simulink model "SWC_VES_type"  (R2021b)
settings: Solver=FixedStepDiscrete  StartTime=0.0  StopTime=10.0  FixedStep=0.001  RelTol=1e-3
undefined symbols (not defined in the file or in its folder): R_HALINCDD_CSOP_IPCF_Handler
libraries: simulink x32
settings Model: DataDictionary=APPTypes.sldd  Creator=FVT23010  LastModifiedBy=FVT23010
settings DataIOCC: SaveFormat=StructureWithTime
settings OptimizationCC: DefaultParameterBehavior=Inlined  EnhancedBackFolding=on  PassReuseOutputArgsAs=Individual arguments  ZeroExternalMemoryAtStartup=off  ZeroInternalMemoryAtStartup=off  OptimizeBlockOrder=speed  DifferentSizesBufferReuse=on  OptimizationCustomize=off  EfficientTunableParamExpr=on
settings DebuggingCC: ParameterTunabilityLossMsg=error
settings HardwareCC: ProdBitPerPointer=32  ProdBitPerSizeT=32  ProdBitPerPtrDiffT=32  ProdLargestAtomicInteger=Long  ProdLargestAtomicFloat=Double  ProdWordSize=32  ProdLongLongMode=on  ProdHWDeviceType=ARM Compatible->ARM Cortex-M
settings ModelReferenceCC: ModelReferenceNumInstancesAllowed=Single
settings SFSimCC: MATLABDynamicMemAlloc=off
settings RTWCC: Description=AUTOSAR  SystemTargetFile=autosar.tlc  GenCodeOnly=on  TemplateMakefile=ert_default_tmf  PortableWordSizes=on
settings CodeAppCC: ForceParamTrailComments=on  IgnoreCustomStorageClasses=off  OperatorAnnotations=on  SimulinkDataObjDesc=on  SFDataObjDesc=on  InsertBlockDesc=on
settings STFCustomTargetCC: TargetLangStandard=C99 (ISO)  MultiwordLength=256  ParMdlRefBuildCompliant=on  CompOptLevelCompliant=on  IncludeMdlTerminateFcn=off  CombineOutputUpdateFcns=on  SuppressErrorStatus=on  ERTCustomFileBanners=on  SupportNonFinite=off  SupportComplex=off  SupportContinuousTime=off  SupportNonInlinedSFcns=off  RemoveResetFunc=on  MATLABClassNameForMDSCustomization=Simulink.SoftwareTarget.ERTCustomization  AutosarCompliant=on  GRTInterface=off  UseToolchainInfoCompliant=on  LookupTableObjectStructAxisOrder=2,1,3,4,...  LUTObjectStructOrderEvenSpacing=Size,Table,Breakpoints  SystemTargetFile=autosar.tlc
settings ERTTargetCC: TargetLangStandard=C99 (ISO)  ConcurrentExecutionCompliant=off  IncludeMdlTerminateFcn=off  SuppressErrorStatus=on  SupportNonFinite=off  SupportComplex=off  ModelStepFunctionPrototypeControlCompliant=off  CPPClassGenCompliant=off  AutosarCompliant=on  LookupTableObjectStructAxisOrder=2,1,3,4,...  LUTObjectStructOrderEvenSpacing=Size,Table,Breakpoints  GenerateASAP2=on  InlinedParameterPlacement=NonHierarchical  ERTCustomFileTemplate=example_file_process.tlc  ConvertIfToSwitch=off  SuppressUnreachableDefaultCases=off  BooleanTrueId=true_MatlabRTW  BooleanFalseId=false_MatlabRTW

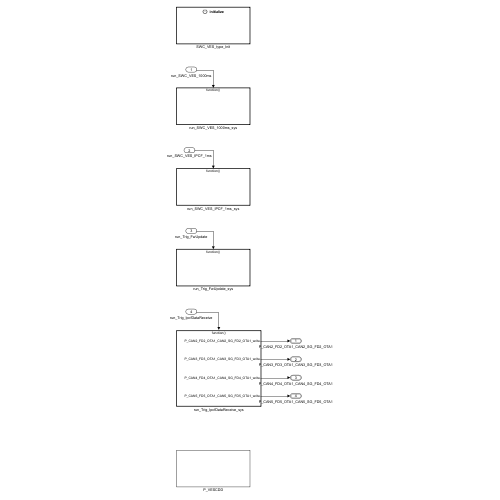
[thumbnail: Simulink's stored preview of the top-level diagram]
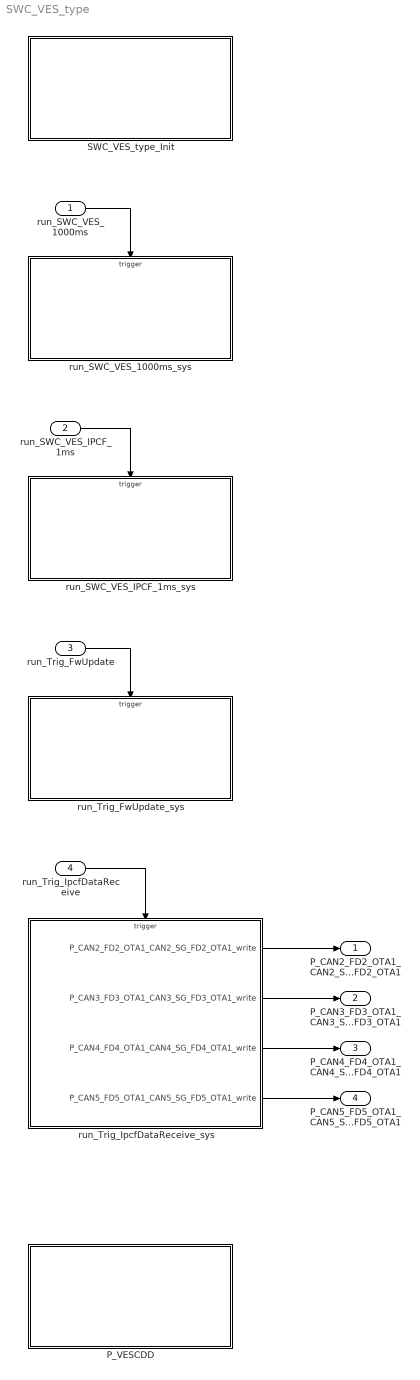
== system SWC_VES_type ==
  run_SWC_VES_1000ms : Inport  SampleTime=1  OutputFunctionCall=on
  run_SWC_VES_IPCF_1ms : Inport  Port=2  SampleTime=0.001  OutputFunctionCall=on
  run_Trig_FwUpdate : Inport  Port=3  OutputFunctionCall=on
  run_Trig_IpcfDataReceive : Inport  Port=4  OutputFunctionCall=on
  P_VESCDD : Subsystem
  SWC_VES_type_Init : Subsystem
  run_SWC_VES_1000ms_sys : Subsystem
  run_SWC_VES_IPCF_1ms_sys : Subsystem
  run_Trig_FwUpdate_sys : Subsystem
  run_Trig_IpcfDataReceive_sys : Subsystem
  P_CAN2_FD2_OTA1_CAN2_SG_FD2_OTA1 : Outport  OutDataTypeStr=Bus: DT_CAN2_SG_FD2_OTA1  PortDimensions=1  BusOutputAsStruct=on
  P_CAN3_FD3_OTA1_CAN3_SG_FD3_OTA1 : Outport  Port=2  OutDataTypeStr=Bus: DT_CAN3_SG_FD3_OTA1  PortDimensions=1  BusOutputAsStruct=on
  P_CAN4_FD4_OTA1_CAN4_SG_FD4_OTA1 : Outport  Port=3  OutDataTypeStr=Bus: DT_CAN4_SG_FD4_OTA1  PortDimensions=1  BusOutputAsStruct=on
  P_CAN5_FD5_OTA1_CAN5_SG_FD5_OTA1 : Outport  Port=4  OutDataTypeStr=Bus: DT_CAN5_SG_FD5_OTA1  PortDimensions=1  BusOutputAsStruct=on
  wires:
  run_Trig_IpcfDataReceive_sys/1(P_CAN2_FD2_OTA1_CAN2_SG_FD2_OTA1_write) -> P_CAN2_FD2_OTA1_CAN2_SG_FD2_OTA1/1
  run_Trig_IpcfDataReceive_sys/2(P_CAN3_FD3_OTA1_CAN3_SG_FD3_OTA1_write) -> P_CAN3_FD3_OTA1_CAN3_SG_FD3_OTA1/1
  run_Trig_IpcfDataReceive_sys/3(P_CAN4_FD4_OTA1_CAN4_SG_FD4_OTA1_write) -> P_CAN4_FD4_OTA1_CAN4_SG_FD4_OTA1/1
  run_Trig_IpcfDataReceive_sys/4(P_CAN5_FD5_OTA1_CAN5_SG_FD5_OTA1_write) -> P_CAN5_FD5_OTA1_CAN5_SG_FD5_OTA1/1
  run_SWC_VES_1000ms/1 -> run_SWC_VES_1000ms_sys/Trigger
  run_SWC_VES_IPCF_1ms/1 -> run_SWC_VES_IPCF_1ms_sys/Trigger
  run_Trig_FwUpdate/1 -> run_Trig_FwUpdate_sys/Trigger
  run_Trig_IpcfDataReceive/1 -> run_Trig_IpcfDataReceive_sys/Trigger

== system SWC_VES_type/P_VESCDD ==
  run_VESCDD_sys : Subsystem

== system SWC_VES_type/SWC_VES_type_Init ==
  Event Listener : EventListener  EventName=reset

== system SWC_VES_type/run_SWC_VES_1000ms_sys ==
  function : TriggerPort  TriggerType=function-call  VariantControl=(inherit)  SampleTimeType=periodic  SampleTime=-1

== system SWC_VES_type/run_SWC_VES_IPCF_1ms_sys ==
  function : TriggerPort  TriggerType=function-call  VariantControl=(inherit)  SampleTimeType=periodic  SampleTime=-1
  R_HALINCDD_CSOP_IPCF_Handler : FunctionCaller  FunctionPrototype=R_HALINCDD_CSOP_IPCF_Handler()

== system SWC_VES_type/run_Trig_FwUpdate_sys ==
  function : TriggerPort  TriggerType=function-call  VariantControl=(inherit)

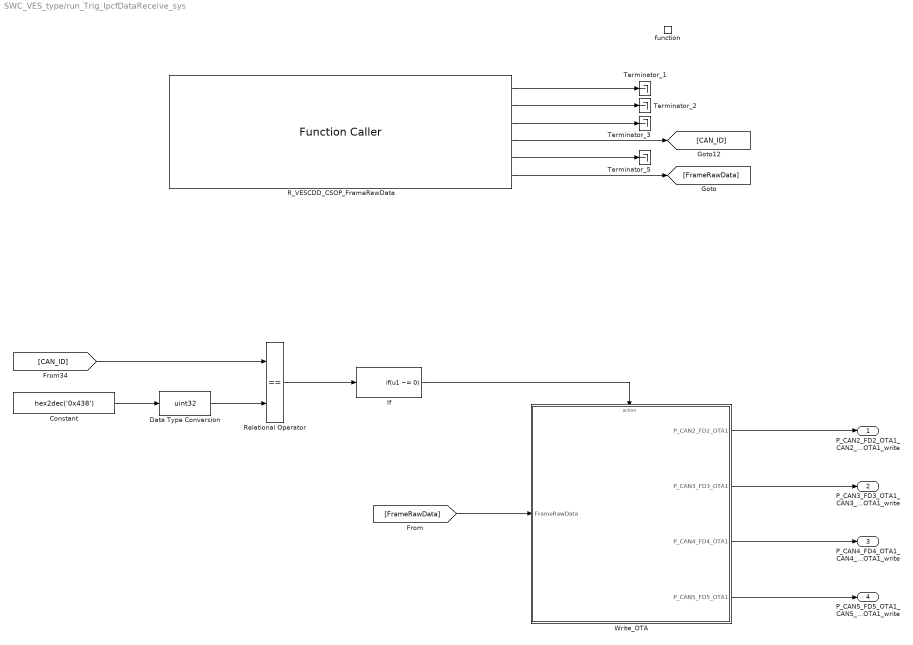
== system SWC_VES_type/run_Trig_IpcfDataReceive_sys ==
  function : TriggerPort  TriggerType=function-call  VariantControl=(inherit)
  Constant : Constant  Value=hex2dec('0x438')
  Data Type Conversion : DataTypeConversion  OutDataTypeStr=uint32
  If : If  IfExpression=u1 ~= 0  ShowElse=off
  R_VESCDD_CSOP_FrameRawData : FunctionCaller  FunctionPrototype=[channel,fd,ext,id,dlc,FrameRawData] = R_VESCDD_CSOP_FrameRawData()  OutputArgumentSpecifications=uint8(1), uint8(1), uint8(1), uint32(1), uint8(1), uint8([1;1;1;1;1;1;1;1;1;1;1;1;1;1;1;1;1;1;1;1;1;1;1;1;1;1;1;1;1;1;1;1;1;1;1;1;1;1;1;1;1;1;1;1;1;1;1;1;1;1;1;1;1;1;1;1;1;1;1;1;1;1;1;1])
  Relational Operator : RelationalOperator  Operator===  OutDataTypeStr=boolean  RndMeth=Simplest
  Terminator_{1..3,5} (4 alike) : Terminator
  Write_OTA : Subsystem  TreatAsAtomicUnit=on
  P_CAN2_FD2_OTA1_CAN2_SG_FD2_OTA1_write : Outport
  P_CAN3_FD3_OTA1_CAN3_SG_FD3_OTA1_write : Outport  Port=2
  P_CAN4_FD4_OTA1_CAN4_SG_FD4_OTA1_write : Outport  Port=3
  P_CAN5_FD5_OTA1_CAN5_SG_FD5_OTA1_write : Outport  Port=4
  wires:
  R_VESCDD_CSOP_FrameRawData/6 -> [FrameRawData]
  R_VESCDD_CSOP_FrameRawData/3 -> Terminator_3/1
  R_VESCDD_CSOP_FrameRawData/5 -> Terminator_5/1
  R_VESCDD_CSOP_FrameRawData/4 -> [CAN_ID]
  R_VESCDD_CSOP_FrameRawData/1 -> Terminator_1/1
  R_VESCDD_CSOP_FrameRawData/2 -> Terminator_2/1
  [FrameRawData] -> Write_OTA/1(FrameRawData)
  Relational Operator/1 -> If/1
  [CAN_ID] -> Relational Operator/1
  Constant/1 -> Data Type Conversion/1
  If/1 -> Write_OTA/Action
  Data Type Conversion/1 -> Relational Operator/2
  Write_OTA/1(P_CAN2_FD2_OTA1) -> P_CAN2_FD2_OTA1_CAN2_SG_FD2_OTA1_write/1
  Write_OTA/2(P_CAN3_FD3_OTA1) -> P_CAN3_FD3_OTA1_CAN3_SG_FD3_OTA1_write/1
  Write_OTA/3(P_CAN4_FD4_OTA1) -> P_CAN4_FD4_OTA1_CAN4_SG_FD4_OTA1_write/1
  Write_OTA/4(P_CAN5_FD5_OTA1) -> P_CAN5_FD5_OTA1_CAN5_SG_FD5_OTA1_write/1

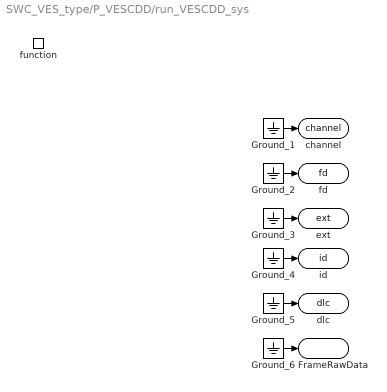
== system SWC_VES_type/P_VESCDD/run_VESCDD_sys ==
  function : TriggerPort  TriggerType=function-call  IsSimulinkFunction=on  FunctionName=run_VESCDD  VariantControl=(inherit)
  Ground_{1..6} (6 alike) : Ground
  channel : ArgOut  OutDataTypeStr=uint8  ArgumentName=channel
  fd : ArgOut  Port=2  OutDataTypeStr=uint8  ArgumentName=fd
  ext : ArgOut  Port=3  OutDataTypeStr=uint8  ArgumentName=ext
  id : ArgOut  Port=4  OutDataTypeStr=uint32  ArgumentName=id
  dlc : ArgOut  Port=5  OutDataTypeStr=uint8  ArgumentName=dlc
  FrameRawData : ArgOut  Port=6  OutDataTypeStr=uint8  PortDimensions=64  ArgumentName=FrameRawData
  wires:
  Ground_1/1 -> channel/1
  Ground_2/1 -> fd/1
  Ground_3/1 -> ext/1
  Ground_4/1 -> id/1
  Ground_5/1 -> dlc/1
  Ground_6/1 -> FrameRawData/1

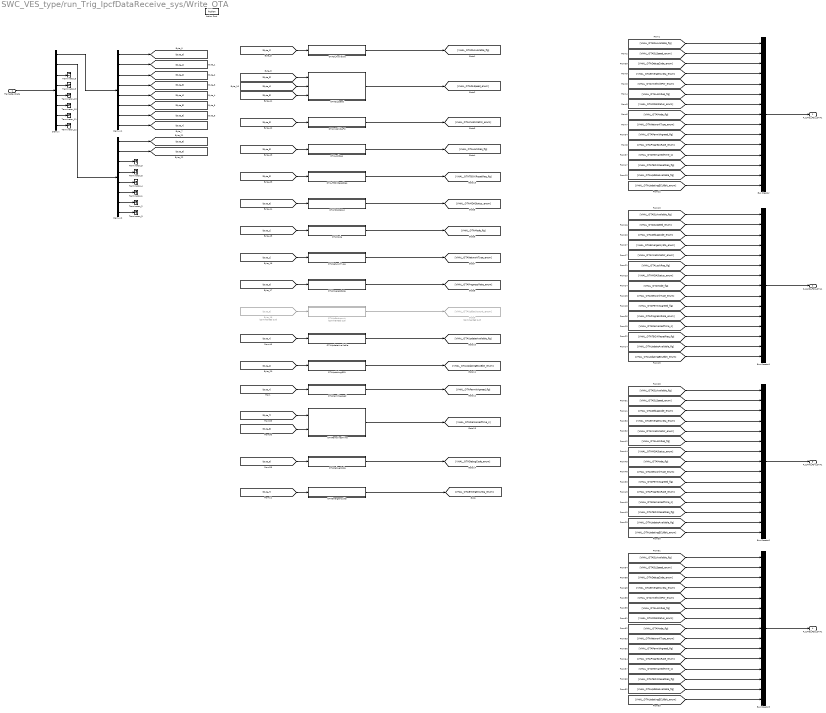
== system SWC_VES_type/run_Trig_IpcfDataReceive_sys/Write_OTA ==
  FrameRawData : Inport
  Action Port : ActionPort  ActionPortLabel=if(u1 ~= 0)
  Bus Creator : BusCreator  Inputs=15  OutDataTypeStr=Bus: DT_CAN2_SG_FD2_OTA1  NonVirtualBus=on
      settings: InheritFromInputs=off
  Bus Creator1 : BusCreator  Inputs=15  OutDataTypeStr=Bus: DT_CAN3_SG_FD3_OTA1  NonVirtualBus=on
      settings: InheritFromInputs=off
  Bus Creator2 : BusCreator  Inputs=15  OutDataTypeStr=Bus: DT_CAN4_SG_FD4_OTA1  NonVirtualBus=on
      settings: InheritFromInputs=off
  Bus Creator3 : BusCreator  Inputs=15  OutDataTypeStr=Bus: DT_CAN5_SG_FD5_OTA1  NonVirtualBus=on
      settings: InheritFromInputs=off
  Byte_18 : From  Commented=on  GotoTag=Byte_6
  Demux : Demux  Outputs=8
  Demux1 : Demux  Outputs=8
  Demux2 : Demux  Outputs=8
  Goto9 : Goto  Commented=on  GotoTag=VHAL_OTAUpBackcount_enum
  OTADLAvailable : Subsystem
  OTADLSpeed : Subsystem
  OTADebugCode : Subsystem
  OTAEmergencySta : Subsystem
  OTAInVehicleFW : Subsystem
  OTALockReq : Subsystem
  OTAMDAStatus : Subsystem
  OTAMode : Subsystem
  OTANetworkType : Subsystem
  OTAPermitAgreed : Subsystem
  OTAProgressRate : Subsystem
  OTARemainedTime : Subsystem
  OTAUpBackcount : Subsystem  Commented=on
  OTAUpdateAvailable : Subsystem
  OTAUpdatingECU : Subsystem
  OTA_TBOXResetReq : Subsystem
  Terminator_{1..6,8..13} (12 alike) : Terminator
  P_CAN2_FD2_OTA1 : Outport
  P_CAN3_FD3_OTA1 : Outport  Port=2
  P_CAN4_FD4_OTA1 : Outport  Port=3
  P_CAN5_FD5_OTA1 : Outport  Port=4
  wires:
  [Byte_2] -> OTAUpdatingECU/1(Byte_2)
  Demux1/7 -> [Byte_6]  "Raw_Byte6"
  Demux1/4 -> [Byte_3]  "Raw_Byte3"
  Demux1/6 -> [Byte_5]  "Raw_Byte5"
  [Byte_5] -> OTADLSpeed/3(Byte_5)
  Demux/1 -> Demux1/1
  [Byte_7] -> OTAUpdateAvailable/1(Byte_7)
  Demux/4 -> Terminator_9/1
  [Byte_3] -> OTALockReq/1(Byte_3)
  [Byte_3] -> OTADLSpeed/1(Byte_3)
  Demux/5 -> Terminator_13/1
  [Byte_4] -> OTADLSpeed/2(Byte_4)
  Byte_18/1 -> OTAUpBackcount/1(Byte_6)
  Demux1/8 -> [Byte_7]  "Raw_Byte7"
  Demux1/3 -> [Byte_2]  "Raw_Byte2"
  Demux1/2 -> [Byte_1]  "Raw_Byte1"
  Demux1/5 -> [Byte_4]  "Raw_Byte4"
  Demux1/1 -> [Byte_0]  "Raw_Byte0"
  [Byte_1] -> OTANetworkType/1(Byte_1)
  Demux/7 -> Terminator_11/1
  FrameRawData/1 -> Demux/1
  [Byte_6] -> OTAMDAStatus/1(Byte_1)
  Demux/3 -> Terminator_8/1
  [Byte_1] -> OTAMode/1(Byte_1)
  [Byte_0] -> OTAProgressRate/1(Byte_0)
  [Byte_3] -> OTAInVehicleFW/1(Byte_3)
  [Byte_1] -> OTADLAvailable/1(Byte_1)
  Demux/8 -> Terminator_12/1
  Demux/6 -> Terminator_10/1
  OTAUpdateAvailable/1(VHAL_OTAUpdateAvailable_flg) -> [VHAL_OTAUpdateAvailable_flg]
  OTAMode/1(VHAL_OTAMode_flg) -> [VHAL_OTAMode_flg]
  OTAInVehicleFW/1(VHAL_OTAInVehicleFW_enum) -> [VHAL_OTAInVehicleFW_enum]
  OTADLAvailable/1(VHAL_OTADLAvailable_flg) -> [VHAL_OTADLAvailable_flg]
  OTANetworkType/1(VHAL_OTANetworkType_enum) -> [VHAL_OTANetworkType_enum]
  OTADLSpeed/1(VHAL_OTADLSpeed_enum) -> [VHAL_OTADLSpeed_enum]
  OTAMDAStatus/1(VHAL_OTAMDAStatus_enum) -> [VHAL_OTAMDAStatus_enum]
  OTAUpdatingECU/1(VHAL_OTAUpdatingECU_enum) -> [VHAL_OTAUpdatingECU8bit_enum]
  OTALockReq/1(VHAL_OTALockReq_flg) -> [VHAL_OTALockReq_flg]
  OTAUpBackcount/1(VHAL_OTAUpBackcount_enum) -> Goto9/1
  OTAProgressRate/1(VHAL_OTAProgressRate_enum) -> [VHAL_OTAProgressRate_enum]
  Demux/2 -> Demux2/1
  Demux2/1 -> [Byte_8]  "Raw_Byte8"
  Demux2/2 -> [Byte_9]  "Raw_Byte9"
  Demux2/3 -> Terminator_5/1
  Demux2/5 -> Terminator_4/1
  Demux2/6 -> Terminator_1/1
  Demux2/7 -> Terminator_2/1
  Demux2/8 -> Terminator_3/1
  [Byte_7] -> OTAPermitAgreed/1(Byte_7)
  OTAPermitAgreed/1(VHAL_OTAPermitAgreed_flg) -> [VHAL_OTAPermitAgreed_flg]
  [Byte_8] -> OTARemainedTime/2(Byte_8)
  [Byte_7] -> OTARemainedTime/1(Byte_7)
  OTARemainedTime/1(VHAL_OTARemainedTime_s) -> [VHAL_OTARemainedTime_s]
  [Byte_9] -> OTADebugCode/1(Byte_9)
  OTADebugCode/1(VHAL_OTADebugCode_enum) -> [VHAL_OTADebugCode_enum]
  [VHAL_OTADLAvailable_flg] -> Bus Creator/1
  [VHAL_OTADebugCode_enum] -> Bus Creator/3
  Bus Creator/1 -> P_CAN2_FD2_OTA1/1
  [VHAL_OTADLSpeed_enum] -> Bus Creator/2
  Demux2/4 -> Terminator_6/1  "Raw_Byte11"
  OTA_TBOXResetReq/1(VHAL_OTALockReq_flg) -> [VHAL_OTATBOXResetReq_flg]
  [Byte_3] -> OTA_TBOXResetReq/1(Byte_3)
  [VHAL_OTAEmergencySta_enum] -> Bus Creator/4
  [VHAL_OTAInVehicleFW_enum] -> Bus Creator/5
  [VHAL_OTALockReq_flg] -> Bus Creator/6
  [VHAL_OTAMDAStatus_enum] -> Bus Creator/7
  [VHAL_OTAMode_flg] -> Bus Creator/8
  [VHAL_OTANetworkType_enum] -> Bus Creator/9
  [VHAL_OTAPermitAgreed_flg] -> Bus Creator/10
  [VHAL_OTAProgressRate_enum] -> Bus Creator/11
  [VHAL_OTARemainedTime_s] -> Bus Creator/12
  [VHAL_OTATBOXResetReq_flg] -> Bus Creator/13
  [VHAL_OTAUpdateAvailable_flg] -> Bus Creator/14
  [VHAL_OTAUpdatingECU8bit_enum] -> Bus Creator/15
  OTAEmergencySta/1(VHAL_OTAEmergencySta_enum) -> [VHAL_OTAEmergencySta_enum]
  [Byte_7] -> OTAEmergencySta/1(Byte_7)
  [VHAL_OTAUpdatingECU8bit_enum] -> Bus Creator1/15
  [VHAL_OTAUpdateAvailable_flg] -> Bus Creator1/14
  [VHAL_OTATBOXResetReq_flg] -> Bus Creator1/13
  [VHAL_OTARemainedTime_s] -> Bus Creator1/12
  [VHAL_OTAProgressRate_enum] -> Bus Creator1/11
  [VHAL_OTAPermitAgreed_flg] -> Bus Creator1/10
  [VHAL_OTANetworkType_enum] -> Bus Creator1/9
  [VHAL_OTAMode_flg] -> Bus Creator1/8
  [VHAL_OTAMDAStatus_enum] -> Bus Creator1/7
  [VHAL_OTALockReq_flg] -> Bus Creator1/6
  [VHAL_OTAInVehicleFW_enum] -> Bus Creator1/5
  [VHAL_OTAEmergencySta_enum] -> Bus Creator1/4
  [VHAL_OTADLSpeed_enum] -> Bus Creator1/2
  Bus Creator1/1 -> P_CAN3_FD3_OTA1/1
  [VHAL_OTADebugCode_enum] -> Bus Creator1/3
  [VHAL_OTADLAvailable_flg] -> Bus Creator1/1
  [VHAL_OTADLAvailable_flg] -> Bus Creator2/1
  [VHAL_OTADebugCode_enum] -> Bus Creator2/3
  Bus Creator2/1 -> P_CAN4_FD4_OTA1/1
  [VHAL_OTADLSpeed_enum] -> Bus Creator2/2
  [VHAL_OTAEmergencySta_enum] -> Bus Creator2/4
  [VHAL_OTAInVehicleFW_enum] -> Bus Creator2/5
  [VHAL_OTALockReq_flg] -> Bus Creator2/6
  [VHAL_OTAMDAStatus_enum] -> Bus Creator2/7
  [VHAL_OTAMode_flg] -> Bus Creator2/8
  [VHAL_OTANetworkType_enum] -> Bus Creator2/9
  [VHAL_OTAPermitAgreed_flg] -> Bus Creator2/10
  [VHAL_OTAProgressRate_enum] -> Bus Creator2/11
  [VHAL_OTARemainedTime_s] -> Bus Creator2/12
  [VHAL_OTATBOXResetReq_flg] -> Bus Creator2/13
  [VHAL_OTAUpdateAvailable_flg] -> Bus Creator2/14
  [VHAL_OTAUpdatingECU8bit_enum] -> Bus Creator2/15
  [VHAL_OTAUpdatingECU8bit_enum] -> Bus Creator3/15
  [VHAL_OTAUpdateAvailable_flg] -> Bus Creator3/14
  [VHAL_OTATBOXResetReq_flg] -> Bus Creator3/13
  [VHAL_OTARemainedTime_s] -> Bus Creator3/12
  [VHAL_OTAProgressRate_enum] -> Bus Creator3/11
  [VHAL_OTAPermitAgreed_flg] -> Bus Creator3/10
  [VHAL_OTANetworkType_enum] -> Bus Creator3/9
  [VHAL_OTAMode_flg] -> Bus Creator3/8
  [VHAL_OTAMDAStatus_enum] -> Bus Creator3/7
  [VHAL_OTALockReq_flg] -> Bus Creator3/6
  [VHAL_OTAInVehicleFW_enum] -> Bus Creator3/5
  [VHAL_OTAEmergencySta_enum] -> Bus Creator3/4
  [VHAL_OTADLSpeed_enum] -> Bus Creator3/2
  Bus Creator3/1 -> P_CAN5_FD5_OTA1/1
  [VHAL_OTADebugCode_enum] -> Bus Creator3/3
  [VHAL_OTADLAvailable_flg] -> Bus Creator3/1

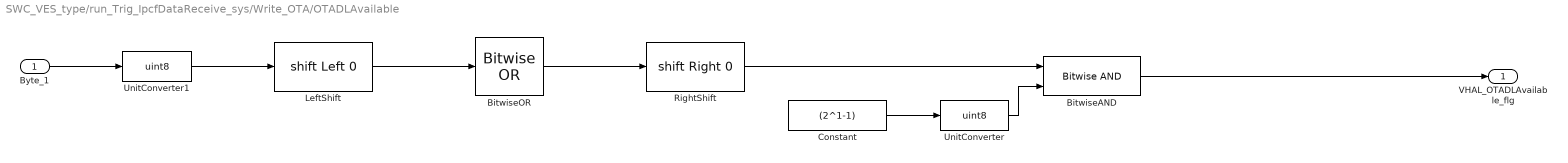
== system SWC_VES_type/run_Trig_IpcfDataReceive_sys/Write_OTA/OTADLAvailable ==
  Byte_1 : Inport
  BitwiseAND : simulink/Logic and Bit Operations/Bitwise Operator  logicop=AND  UseBitMask=off  NumInputPorts=2  BitMask=bin2dec('11011001')  BitMaskRealWorld=Stored Integer
  BitwiseOR : simulink/Logic and Bit Operations/Bitwise Operator  logicop=OR  UseBitMask=off  BitMask=bin2dec('11011001')  BitMaskRealWorld=Stored Integer
  Constant : Constant  Value=(2^1-1)
  LeftShift : ArithShift  BitShiftDirection=Left
  RightShift : ArithShift  BitShiftDirection=Right
  UnitConverter : DataTypeConversion  OutDataTypeStr=uint8
  UnitConverter1 : DataTypeConversion  OutDataTypeStr=uint8
  VHAL_OTADLAvailable_flg : Outport
  wires:
  BitwiseOR/1 -> RightShift/1
  RightShift/1 -> BitwiseAND/1
  UnitConverter/1 -> BitwiseAND/2
  Constant/1 -> UnitConverter/1
  BitwiseAND/1 -> VHAL_OTADLAvailable_flg/1
  LeftShift/1 -> BitwiseOR/1
  UnitConverter1/1 -> LeftShift/1
  Byte_1/1 -> UnitConverter1/1

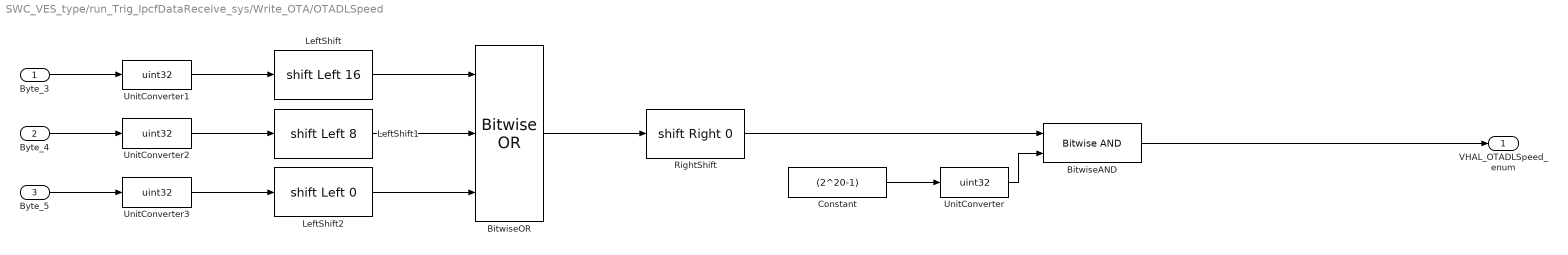
== system SWC_VES_type/run_Trig_IpcfDataReceive_sys/Write_OTA/OTADLSpeed ==
  Byte_3 : Inport
  Byte_4 : Inport  Port=2
  Byte_5 : Inport  Port=3
  BitwiseAND : simulink/Logic and Bit Operations/Bitwise Operator  logicop=AND  UseBitMask=off  NumInputPorts=2  BitMask=bin2dec('11011001')  BitMaskRealWorld=Stored Integer
  BitwiseOR : simulink/Logic and Bit Operations/Bitwise Operator  logicop=OR  UseBitMask=off  NumInputPorts=3  BitMask=bin2dec('11011001')  BitMaskRealWorld=Stored Integer
  Constant : Constant  Value=(2^20-1)
  LeftShift : ArithShift  BitShiftNumber=16  BitShiftDirection=Left
  LeftShift1 : ArithShift  BitShiftNumber=8  BitShiftDirection=Left
  LeftShift2 : ArithShift  BitShiftDirection=Left
  RightShift : ArithShift  BitShiftDirection=Right
  UnitConverter{,1..3} (4 alike) : DataTypeConversion  OutDataTypeStr=uint32
  VHAL_OTADLSpeed_enum : Outport
  wires:
  BitwiseOR/1 -> RightShift/1
  RightShift/1 -> BitwiseAND/1
  UnitConverter/1 -> BitwiseAND/2
  Constant/1 -> UnitConverter/1
  BitwiseAND/1 -> VHAL_OTADLSpeed_enum/1
  LeftShift/1 -> BitwiseOR/1
  UnitConverter1/1 -> LeftShift/1
  Byte_3/1 -> UnitConverter1/1
  LeftShift1/1 -> BitwiseOR/2
  UnitConverter2/1 -> LeftShift1/1
  Byte_4/1 -> UnitConverter2/1
  LeftShift2/1 -> BitwiseOR/3
  UnitConverter3/1 -> LeftShift2/1
  Byte_5/1 -> UnitConverter3/1

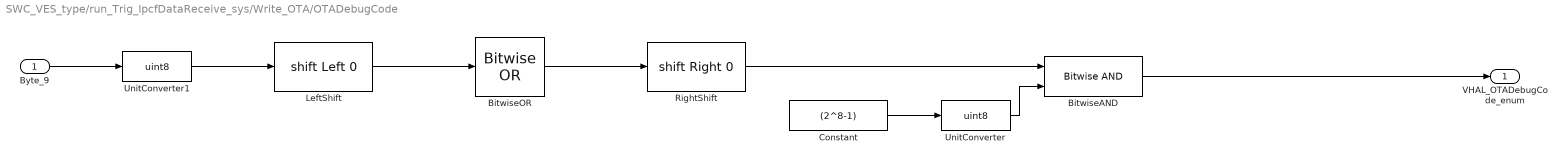
== system SWC_VES_type/run_Trig_IpcfDataReceive_sys/Write_OTA/OTADebugCode ==
  Byte_9 : Inport
  BitwiseAND : simulink/Logic and Bit Operations/Bitwise Operator  logicop=AND  UseBitMask=off  NumInputPorts=2  BitMask=bin2dec('11011001')  BitMaskRealWorld=Stored Integer
  BitwiseOR : simulink/Logic and Bit Operations/Bitwise Operator  logicop=OR  UseBitMask=off  BitMask=bin2dec('11011001')  BitMaskRealWorld=Stored Integer
  Constant : Constant  Value=(2^8-1)
  LeftShift : ArithShift  BitShiftDirection=Left
  RightShift : ArithShift  BitShiftDirection=Right
  UnitConverter : DataTypeConversion  OutDataTypeStr=uint8
  UnitConverter1 : DataTypeConversion  OutDataTypeStr=uint8
  VHAL_OTADebugCode_enum : Outport
  wires:
  BitwiseOR/1 -> RightShift/1
  RightShift/1 -> BitwiseAND/1
  UnitConverter/1 -> BitwiseAND/2
  Constant/1 -> UnitConverter/1
  BitwiseAND/1 -> VHAL_OTADebugCode_enum/1
  LeftShift/1 -> BitwiseOR/1
  UnitConverter1/1 -> LeftShift/1
  Byte_9/1 -> UnitConverter1/1

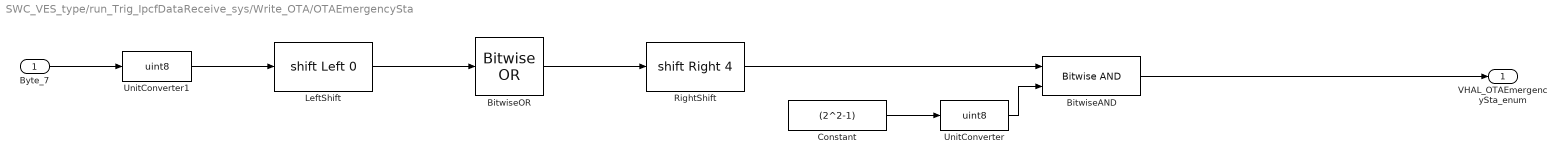
== system SWC_VES_type/run_Trig_IpcfDataReceive_sys/Write_OTA/OTAEmergencySta ==
  Byte_7 : Inport
  BitwiseAND : simulink/Logic and Bit Operations/Bitwise Operator  logicop=AND  UseBitMask=off  NumInputPorts=2  BitMask=bin2dec('11011001')  BitMaskRealWorld=Stored Integer
  BitwiseOR : simulink/Logic and Bit Operations/Bitwise Operator  logicop=OR  UseBitMask=off  BitMask=bin2dec('11011001')  BitMaskRealWorld=Stored Integer
  Constant : Constant  Value=(2^2-1)
  LeftShift : ArithShift  BitShiftDirection=Left
  RightShift : ArithShift  BitShiftNumber=4  BitShiftDirection=Right
  UnitConverter : DataTypeConversion  OutDataTypeStr=uint8
  UnitConverter1 : DataTypeConversion  OutDataTypeStr=uint8
  VHAL_OTAEmergencySta_enum : Outport
  wires:
  Byte_7/1 -> UnitConverter1/1
  UnitConverter1/1 -> LeftShift/1
  LeftShift/1 -> BitwiseOR/1
  BitwiseAND/1 -> VHAL_OTAEmergencySta_enum/1
  Constant/1 -> UnitConverter/1
  UnitConverter/1 -> BitwiseAND/2
  RightShift/1 -> BitwiseAND/1
  BitwiseOR/1 -> RightShift/1

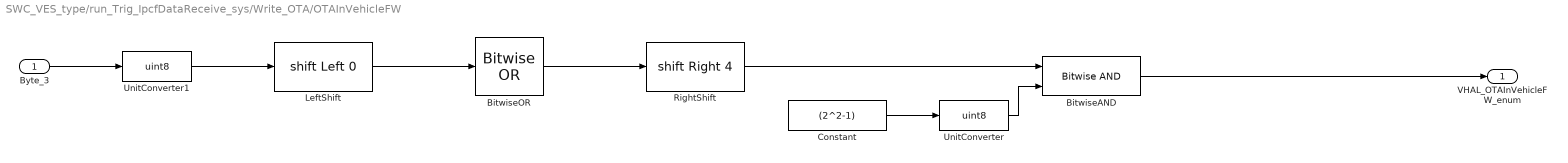
== system SWC_VES_type/run_Trig_IpcfDataReceive_sys/Write_OTA/OTAInVehicleFW ==
  Byte_3 : Inport
  BitwiseAND : simulink/Logic and Bit Operations/Bitwise Operator  logicop=AND  UseBitMask=off  NumInputPorts=2  BitMask=bin2dec('11011001')  BitMaskRealWorld=Stored Integer
  BitwiseOR : simulink/Logic and Bit Operations/Bitwise Operator  logicop=OR  UseBitMask=off  BitMask=bin2dec('11011001')  BitMaskRealWorld=Stored Integer
  Constant : Constant  Value=(2^2-1)
  LeftShift : ArithShift  BitShiftDirection=Left
  RightShift : ArithShift  BitShiftNumber=4  BitShiftDirection=Right
  UnitConverter : DataTypeConversion  OutDataTypeStr=uint8
  UnitConverter1 : DataTypeConversion  OutDataTypeStr=uint8
  VHAL_OTAInVehicleFW_enum : Outport
  wires:
  BitwiseOR/1 -> RightShift/1
  RightShift/1 -> BitwiseAND/1
  UnitConverter/1 -> BitwiseAND/2
  Constant/1 -> UnitConverter/1
  BitwiseAND/1 -> VHAL_OTAInVehicleFW_enum/1
  LeftShift/1 -> BitwiseOR/1
  UnitConverter1/1 -> LeftShift/1
  Byte_3/1 -> UnitConverter1/1

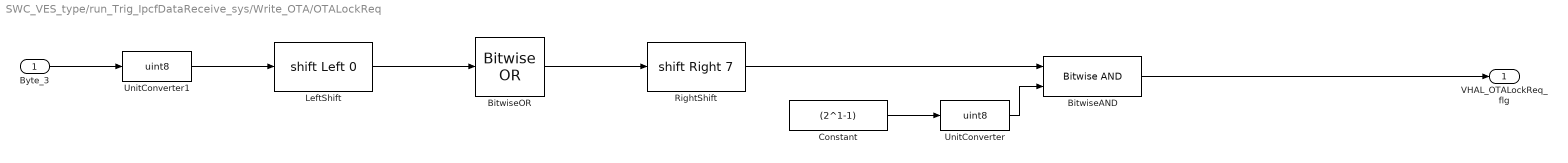
== system SWC_VES_type/run_Trig_IpcfDataReceive_sys/Write_OTA/OTALockReq ==
  Byte_3 : Inport
  BitwiseAND : simulink/Logic and Bit Operations/Bitwise Operator  logicop=AND  UseBitMask=off  NumInputPorts=2  BitMask=bin2dec('11011001')  BitMaskRealWorld=Stored Integer
  BitwiseOR : simulink/Logic and Bit Operations/Bitwise Operator  logicop=OR  UseBitMask=off  BitMask=bin2dec('11011001')  BitMaskRealWorld=Stored Integer
  Constant : Constant  Value=(2^1-1)
  LeftShift : ArithShift  BitShiftDirection=Left
  RightShift : ArithShift  BitShiftNumber=7  BitShiftDirection=Right
  UnitConverter : DataTypeConversion  OutDataTypeStr=uint8
  UnitConverter1 : DataTypeConversion  OutDataTypeStr=uint8
  VHAL_OTALockReq_flg : Outport
  wires:
  BitwiseOR/1 -> RightShift/1
  RightShift/1 -> BitwiseAND/1
  UnitConverter/1 -> BitwiseAND/2
  Constant/1 -> UnitConverter/1
  BitwiseAND/1 -> VHAL_OTALockReq_flg/1
  LeftShift/1 -> BitwiseOR/1
  UnitConverter1/1 -> LeftShift/1
  Byte_3/1 -> UnitConverter1/1

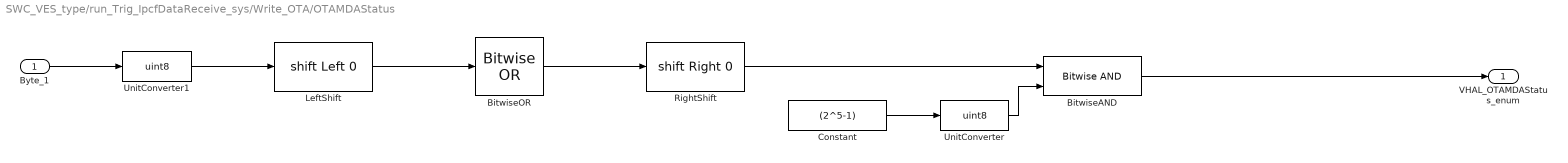
== system SWC_VES_type/run_Trig_IpcfDataReceive_sys/Write_OTA/OTAMDAStatus ==
  Byte_1 : Inport
  BitwiseAND : simulink/Logic and Bit Operations/Bitwise Operator  logicop=AND  UseBitMask=off  NumInputPorts=2  BitMask=bin2dec('11011001')  BitMaskRealWorld=Stored Integer
  BitwiseOR : simulink/Logic and Bit Operations/Bitwise Operator  logicop=OR  UseBitMask=off  BitMask=bin2dec('11011001')  BitMaskRealWorld=Stored Integer
  Constant : Constant  Value=(2^5-1)
  LeftShift : ArithShift  BitShiftDirection=Left
  RightShift : ArithShift  BitShiftDirection=Right
  UnitConverter : DataTypeConversion  OutDataTypeStr=uint8
  UnitConverter1 : DataTypeConversion  OutDataTypeStr=uint8
  VHAL_OTAMDAStatus_enum : Outport
  wires:
  BitwiseOR/1 -> RightShift/1
  RightShift/1 -> BitwiseAND/1
  UnitConverter/1 -> BitwiseAND/2
  Constant/1 -> UnitConverter/1
  BitwiseAND/1 -> VHAL_OTAMDAStatus_enum/1
  LeftShift/1 -> BitwiseOR/1
  UnitConverter1/1 -> LeftShift/1
  Byte_1/1 -> UnitConverter1/1

== system SWC_VES_type/run_Trig_IpcfDataReceive_sys/Write_OTA/OTAMode ==
  Byte_1 : Inport
  BitwiseAND : simulink/Logic and Bit Operations/Bitwise Operator  logicop=AND  UseBitMask=off  NumInputPorts=2  BitMask=bin2dec('11011001')  BitMaskRealWorld=Stored Integer
  BitwiseOR : simulink/Logic and Bit Operations/Bitwise Operator  logicop=OR  UseBitMask=off  BitMask=bin2dec('11011001')  BitMaskRealWorld=Stored Integer
  Constant : Constant  Value=(2^1-1)
  LeftShift : ArithShift  BitShiftDirection=Left
  RightShift : ArithShift  BitShiftNumber=1  BitShiftDirection=Right
  UnitConverter : DataTypeConversion  OutDataTypeStr=uint8
  UnitConverter1 : DataTypeConversion  OutDataTypeStr=uint8
  VHAL_OTAMode_flg : Outport
  wires:
  BitwiseOR/1 -> RightShift/1
  RightShift/1 -> BitwiseAND/1
  UnitConverter/1 -> BitwiseAND/2
  Constant/1 -> UnitConverter/1
  BitwiseAND/1 -> VHAL_OTAMode_flg/1
  LeftShift/1 -> BitwiseOR/1
  UnitConverter1/1 -> LeftShift/1
  Byte_1/1 -> UnitConverter1/1

== system SWC_VES_type/run_Trig_IpcfDataReceive_sys/Write_OTA/OTANetworkType ==
  Byte_1 : Inport
  BitwiseAND : simulink/Logic and Bit Operations/Bitwise Operator  logicop=AND  UseBitMask=off  NumInputPorts=2  BitMask=bin2dec('11011001')  BitMaskRealWorld=Stored Integer
  BitwiseOR : simulink/Logic and Bit Operations/Bitwise Operator  logicop=OR  UseBitMask=off  BitMask=bin2dec('11011001')  BitMaskRealWorld=Stored Integer
  Constant : Constant  Value=(2^2-1)
  LeftShift : ArithShift  BitShiftDirection=Left
  RightShift : ArithShift  BitShiftNumber=2  BitShiftDirection=Right
  UnitConverter : DataTypeConversion  OutDataTypeStr=uint8
  UnitConverter1 : DataTypeConversion  OutDataTypeStr=uint8
  VHAL_OTANetworkType_enum : Outport
  wires:
  BitwiseOR/1 -> RightShift/1
  RightShift/1 -> BitwiseAND/1
  UnitConverter/1 -> BitwiseAND/2
  Constant/1 -> UnitConverter/1
  BitwiseAND/1 -> VHAL_OTANetworkType_enum/1
  LeftShift/1 -> BitwiseOR/1
  UnitConverter1/1 -> LeftShift/1
  Byte_1/1 -> UnitConverter1/1

== system SWC_VES_type/run_Trig_IpcfDataReceive_sys/Write_OTA/OTAPermitAgreed ==
  Byte_7 : Inport
  BitwiseAND : simulink/Logic and Bit Operations/Bitwise Operator  logicop=AND  UseBitMask=off  NumInputPorts=2  BitMask=bin2dec('11011001')  BitMaskRealWorld=Stored Integer
  BitwiseOR : simulink/Logic and Bit Operations/Bitwise Operator  logicop=OR  UseBitMask=off  BitMask=bin2dec('11011001')  BitMaskRealWorld=Stored Integer
  Constant : Constant  Value=(2^1-1)
  LeftShift : ArithShift  BitShiftDirection=Left
  RightShift : ArithShift  BitShiftNumber=7  BitShiftDirection=Right
  UnitConverter : DataTypeConversion  OutDataTypeStr=uint8
  UnitConverter1 : DataTypeConversion  OutDataTypeStr=uint8
  VHAL_OTAPermitAgreed_flg : Outport
  wires:
  Byte_7/1 -> UnitConverter1/1
  UnitConverter1/1 -> LeftShift/1
  LeftShift/1 -> BitwiseOR/1
  BitwiseAND/1 -> VHAL_OTAPermitAgreed_flg/1
  Constant/1 -> UnitConverter/1
  UnitConverter/1 -> BitwiseAND/2
  RightShift/1 -> BitwiseAND/1
  BitwiseOR/1 -> RightShift/1

== system SWC_VES_type/run_Trig_IpcfDataReceive_sys/Write_OTA/OTAProgressRate ==
  Byte_0 : Inport
  BitwiseAND : simulink/Logic and Bit Operations/Bitwise Operator  logicop=AND  UseBitMask=off  NumInputPorts=2  BitMask=bin2dec('11011001')  BitMaskRealWorld=Stored Integer
  BitwiseOR : simulink/Logic and Bit Operations/Bitwise Operator  logicop=OR  UseBitMask=off  BitMask=bin2dec('11011001')  BitMaskRealWorld=Stored Integer
  Constant : Constant  Value=(2^8-1)
  LeftShift : ArithShift  BitShiftDirection=Left
  RightShift : ArithShift  BitShiftDirection=Right
  UnitConverter : DataTypeConversion  OutDataTypeStr=uint8
  UnitConverter1 : DataTypeConversion  OutDataTypeStr=uint8
  VHAL_OTAProgressRate_enum : Outport
  wires:
  BitwiseOR/1 -> RightShift/1
  RightShift/1 -> BitwiseAND/1
  UnitConverter/1 -> BitwiseAND/2
  Constant/1 -> UnitConverter/1
  BitwiseAND/1 -> VHAL_OTAProgressRate_enum/1
  LeftShift/1 -> BitwiseOR/1
  UnitConverter1/1 -> LeftShift/1
  Byte_0/1 -> UnitConverter1/1

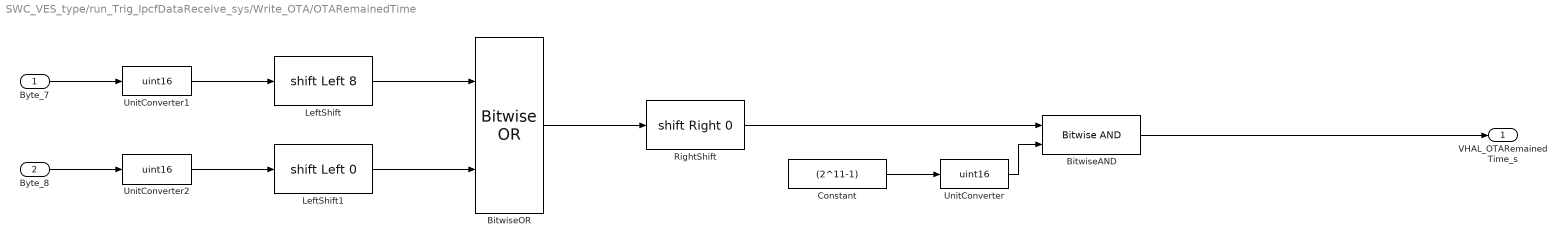
== system SWC_VES_type/run_Trig_IpcfDataReceive_sys/Write_OTA/OTARemainedTime ==
  Byte_7 : Inport
  Byte_8 : Inport  Port=2
  BitwiseAND : simulink/Logic and Bit Operations/Bitwise Operator  logicop=AND  UseBitMask=off  NumInputPorts=2  BitMask=bin2dec('11011001')  BitMaskRealWorld=Stored Integer
  BitwiseOR : simulink/Logic and Bit Operations/Bitwise Operator  logicop=OR  UseBitMask=off  NumInputPorts=2  BitMask=bin2dec('11011001')  BitMaskRealWorld=Stored Integer
  Constant : Constant  Value=(2^11-1)
  LeftShift : ArithShift  BitShiftNumber=8  BitShiftDirection=Left
  LeftShift1 : ArithShift  BitShiftDirection=Left
  RightShift : ArithShift  BitShiftDirection=Right
  UnitConverter : DataTypeConversion  OutDataTypeStr=uint16
  UnitConverter1 : DataTypeConversion  OutDataTypeStr=uint16
  UnitConverter2 : DataTypeConversion  OutDataTypeStr=uint16
  VHAL_OTARemainedTime_s : Outport
  wires:
  Byte_8/1 -> UnitConverter2/1
  UnitConverter2/1 -> LeftShift1/1
  LeftShift1/1 -> BitwiseOR/2
  Byte_7/1 -> UnitConverter1/1
  UnitConverter1/1 -> LeftShift/1
  LeftShift/1 -> BitwiseOR/1
  BitwiseAND/1 -> VHAL_OTARemainedTime_s/1
  Constant/1 -> UnitConverter/1
  UnitConverter/1 -> BitwiseAND/2
  RightShift/1 -> BitwiseAND/1
  BitwiseOR/1 -> RightShift/1

== system SWC_VES_type/run_Trig_IpcfDataReceive_sys/Write_OTA/OTAUpBackcount ==
  Byte_6 : Inport
  BitwiseAND : simulink/Logic and Bit Operations/Bitwise Operator  logicop=AND  UseBitMask=off  NumInputPorts=2  BitMask=bin2dec('11011001')  BitMaskRealWorld=Stored Integer
  BitwiseOR : simulink/Logic and Bit Operations/Bitwise Operator  logicop=OR  UseBitMask=off  BitMask=bin2dec('11011001')  BitMaskRealWorld=Stored Integer
  Constant : Constant  Value=(2^8-1)
  LeftShift : ArithShift  BitShiftDirection=Left
  RightShift : ArithShift  BitShiftDirection=Right
  UnitConverter : DataTypeConversion  OutDataTypeStr=uint8
  UnitConverter1 : DataTypeConversion  OutDataTypeStr=uint8
  VHAL_OTAUpBackcount_enum : Outport
  wires:
  BitwiseOR/1 -> RightShift/1
  RightShift/1 -> BitwiseAND/1
  UnitConverter/1 -> BitwiseAND/2
  Constant/1 -> UnitConverter/1
  BitwiseAND/1 -> VHAL_OTAUpBackcount_enum/1
  LeftShift/1 -> BitwiseOR/1
  UnitConverter1/1 -> LeftShift/1
  Byte_6/1 -> UnitConverter1/1

== system SWC_VES_type/run_Trig_IpcfDataReceive_sys/Write_OTA/OTAUpdateAvailable ==
  Byte_7 : Inport
  BitwiseAND : simulink/Logic and Bit Operations/Bitwise Operator  logicop=AND  UseBitMask=off  NumInputPorts=2  BitMask=bin2dec('11011001')  BitMaskRealWorld=Stored Integer
  BitwiseOR : simulink/Logic and Bit Operations/Bitwise Operator  logicop=OR  UseBitMask=off  BitMask=bin2dec('11011001')  BitMaskRealWorld=Stored Integer
  Constant : Constant  Value=(2^1-1)
  LeftShift : ArithShift  BitShiftDirection=Left
  RightShift : ArithShift  BitShiftNumber=6  BitShiftDirection=Right
  UnitConverter : DataTypeConversion  OutDataTypeStr=uint8
  UnitConverter1 : DataTypeConversion  OutDataTypeStr=uint8
  VHAL_OTAUpdateAvailable_flg : Outport
  wires:
  BitwiseOR/1 -> RightShift/1
  RightShift/1 -> BitwiseAND/1
  UnitConverter/1 -> BitwiseAND/2
  Constant/1 -> UnitConverter/1
  BitwiseAND/1 -> VHAL_OTAUpdateAvailable_flg/1
  LeftShift/1 -> BitwiseOR/1
  UnitConverter1/1 -> LeftShift/1
  Byte_7/1 -> UnitConverter1/1

== system SWC_VES_type/run_Trig_IpcfDataReceive_sys/Write_OTA/OTAUpdatingECU ==
  Byte_2 : Inport
  BitwiseAND : simulink/Logic and Bit Operations/Bitwise Operator  logicop=AND  UseBitMask=off  NumInputPorts=2  BitMask=bin2dec('11011001')  BitMaskRealWorld=Stored Integer
  BitwiseOR : simulink/Logic and Bit Operations/Bitwise Operator  logicop=OR  UseBitMask=off  BitMask=bin2dec('11011001')  BitMaskRealWorld=Stored Integer
  Constant : Constant  Value=(2^8-1)
  LeftShift : ArithShift  BitShiftDirection=Left
  RightShift : ArithShift  BitShiftDirection=Right
  UnitConverter : DataTypeConversion  OutDataTypeStr=uint8
  UnitConverter1 : DataTypeConversion  OutDataTypeStr=uint8
  VHAL_OTAUpdatingECU_enum : Outport
  wires:
  BitwiseOR/1 -> RightShift/1
  RightShift/1 -> BitwiseAND/1
  UnitConverter/1 -> BitwiseAND/2
  Constant/1 -> UnitConverter/1
  BitwiseAND/1 -> VHAL_OTAUpdatingECU_enum/1
  LeftShift/1 -> BitwiseOR/1
  UnitConverter1/1 -> LeftShift/1
  Byte_2/1 -> UnitConverter1/1

== system SWC_VES_type/run_Trig_IpcfDataReceive_sys/Write_OTA/OTA_TBOXResetReq ==
  Byte_3 : Inport
  BitwiseAND : simulink/Logic and Bit Operations/Bitwise Operator  logicop=AND  UseBitMask=off  NumInputPorts=2  BitMask=bin2dec('11011001')  BitMaskRealWorld=Stored Integer
  BitwiseOR : simulink/Logic and Bit Operations/Bitwise Operator  logicop=OR  UseBitMask=off  BitMask=bin2dec('11011001')  BitMaskRealWorld=Stored Integer
  Constant : Constant  Value=(2^1-1)
  LeftShift : ArithShift  BitShiftDirection=Left
  RightShift : ArithShift  BitShiftNumber=6  BitShiftDirection=Right
  UnitConverter : DataTypeConversion  OutDataTypeStr=uint8
  UnitConverter1 : DataTypeConversion  OutDataTypeStr=uint8
  VHAL_OTALockReq_flg : Outport
  wires:
  Byte_3/1 -> UnitConverter1/1
  UnitConverter1/1 -> LeftShift/1
  LeftShift/1 -> BitwiseOR/1
  BitwiseAND/1 -> VHAL_OTALockReq_flg/1
  Constant/1 -> UnitConverter/1
  UnitConverter/1 -> BitwiseAND/2
  RightShift/1 -> BitwiseAND/1
  BitwiseOR/1 -> RightShift/1
